simulink model "small_square_wave"  (R2014b)
settings: Solver=FixedStepDiscrete  StartTime=0.0  StopTime=inf  FixedStep=0.0005  RelTol=1e-3
StartFcn:
  | tg.sampletime = correctedSampleTime;
undefined symbols (not defined in the file or in its folder): sample_time
settings Model: SimulationMode=external  BufferReuse=off  Creator=wmartin  LastModifiedBy=drl
settings SolverCC: EnableConcurrentExecution=on
settings DataIOCC: LimitDataPoints=off  MaxDataPoints=1e7  SaveFormat=StructureWithTime  SignalLogging=off  DSMLogging=off
settings OptimizationCC: BlockReduction=off  OptimizeBlockIOStorage=off  BufferReuse=off  GlobalBufferReuse=off  ExpressionFolding=off  ExpressionDepthLimit=2147483647  LocalBlockOutputs=off  SimCompilerOptimization=On
settings DebuggingCC: UnderspecifiedInitializationDetection=Classic  MergeDetectMultiDrivingBlocksExec=none  StateNameClashWarn=warning
settings HardwareCC: ProdIntDivRoundTo=Zero  ProdEndianess=LittleEndian  ProdLongLongMode=on  ProdHWDeviceType=Generic->32-bit x86 compatible
settings ModelReferenceCC: UpdateModelReferenceTargets=IfOutOfDate  ModelReferenceNumInstancesAllowed=Single  ModelReferenceMinAlgLoopOccurrences=on
settings RTWCC: SystemTargetFile=slrt.tlc  TemplateMakefile=slrt_default_tmf  Description=Simulink Real-Time  RTWVerbose=off  ProcessScript=slrt_make_rtw_hook  RTWCompilerOptimization=On
settings CodeAppCC: MaxIdLength=256
settings SimulinkRealTimeCC: GeneratePreprocessorConditionals=Disable all  EnableShiftOperators=on  RL32LogBufSizeModifier=1e8

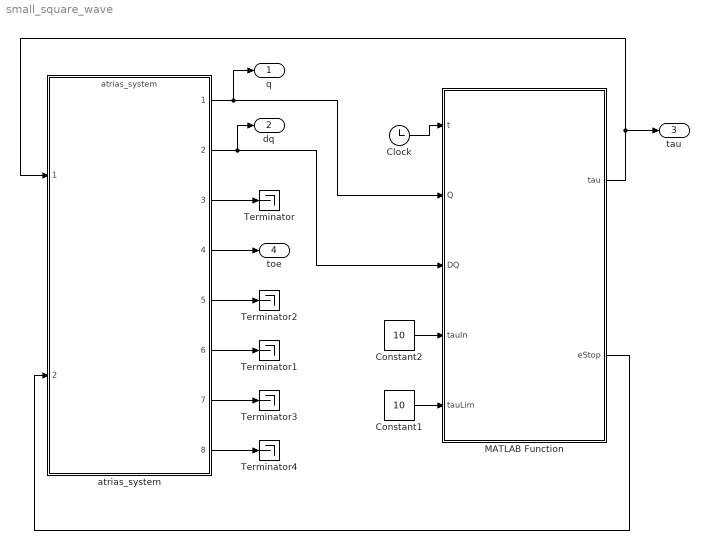
== system small_square_wave ==
  Clock : Clock
  Constant1 : Constant  Value=10
  Constant2 : Constant  Value=10
  MATLAB Function : MATLAB Function  TreatAsAtomicUnit=on  SystemSampleTime=sample_time
  Terminator{,1..4} (5 alike) : Terminator
  atrias_system : ModelReference  ModelNameDialog=atrias_system.slx  SimulationMode=Normal  ModelReferenceVersion=1.2413  CopyOfModelName=atrias_system.slx  DefaultDataLogging=on
  q : Outport
  dq : Outport  Port=2
  tau : Outport  Port=3
  toe : Outport  Port=4
  wires:
  atrias_system/2 -> dq/1, MATLAB Function/3(DQ)
  MATLAB Function/1(tau) -> tau/1, atrias_system/1
  MATLAB Function/2(eStop) -> atrias_system/2
  atrias_system/1 -> q/1, MATLAB Function/2(Q)
  Constant1/1 -> MATLAB Function/5(tauLim)
  atrias_system/3 -> Terminator/1
  atrias_system/4 -> toe/1
  atrias_system/6 -> Terminator1/1
  atrias_system/7 -> Terminator3/1
  atrias_system/5 -> Terminator2/1
  atrias_system/8 -> Terminator4/1
  Clock/1 -> MATLAB Function/1(t)
  Constant2/1 -> MATLAB Function/4(tauIn)

== matlab function small_square_wave/MATLAB Function ==
  data: t input; Q input; DQ input; tauIn input; tau output; eStop output; tauLim input
function [tau, eStop] = smallSquareWave(t, Q, DQ, tauIn, tauLim)
% Description:
%
% Notes:
% 	- State indexes (rBl rBm rAl rAm lBl lBm lAl lAm rHm lHm bR bY bP) 
%   - Input indexes (rB rA rH lB lA lH)
    
    % Generate a small square wave with a period of 100 ms and length of 5
    % ms
    if mod(t,0.1) <= 0.005
        u = tauIn;
    else
        u = 0;
    end
    % Output vector
    tauTemp = [u u 0 u u 0];
    
    % Set default emergency stop to false
    eStop = false;
    
    % Limit torques to be cautious
	tau = clamp(tauTemp, -tauLim, tauLim);

end % sampleController

function b = clamp(a, lim1, lim2)
%CLAMP Clamp value between two values.
	
	% Find which limit is min and max
	aMin = min(lim1, lim2);
	aMax = max(lim1, lim2);

	% Clamp value between limits
	b = max(min(a, aMax), aMin);
end % clamp
